simulink model "gm_HARDWARE_FRIENDLY_FSK"  (R2024a)
settings: Solver=FixedStepDiscrete  StartTime=0.0  StopTime=3.5/B  FixedStep=1/fclk  RelTol=1e-3
undefined symbols (not defined in the file or in its folder): B, DiscIntNeverNeededParam, f0, fclk
libraries: hdlsllib x3, dsphdlsigops2 x2, simulink x1
settings Model: Creator=pc  LastModifiedBy=pc
settings OptimizationCC: BlockReduction=off  ConditionallyExecuteInputs=off
settings DebuggingCC: InheritedTsInSrcMsg=none

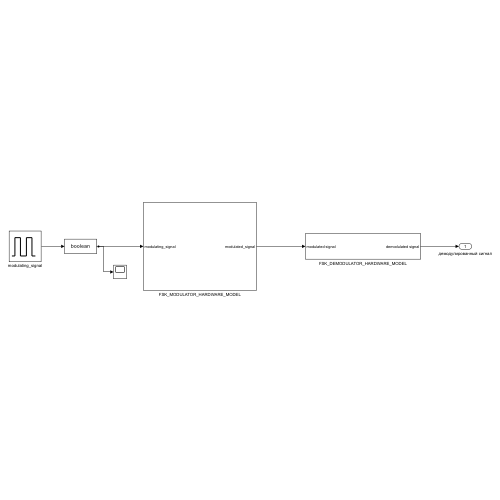
[thumbnail: Simulink's stored preview of the top-level diagram]
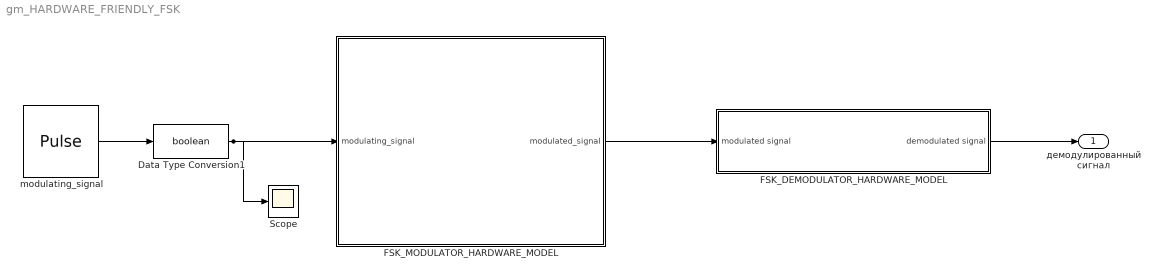
== system gm_HARDWARE_FRIENDLY_FSK ==
  Data Type Conversion1 : DataTypeConversion  OutDataTypeStr=boolean  SaturateOnIntegerOverflow=off  RndMeth=Floor
  FSK_DEMODULATOR_HARDWARE_MODEL : Subsystem
  FSK_MODULATOR_HARDWARE_MODEL : Subsystem
  Scope : Scope
  modulating_signal : DiscretePulseGenerator  PulseType=Time based  Period=2/B  PulseWidth=50
  демодулированный сигнал : Outport
  wires:
  modulating_signal/1 -> Data Type Conversion1/1
  Data Type Conversion1/1 -> FSK_MODULATOR_HARDWARE_MODEL/1(modulating_signal), Scope/1
  FSK_DEMODULATOR_HARDWARE_MODEL/1(demodulated signal) -> демодулированный сигнал/1
  FSK_MODULATOR_HARDWARE_MODEL/1(modulated_signal) -> FSK_DEMODULATOR_HARDWARE_MODEL/1(modulated signal)

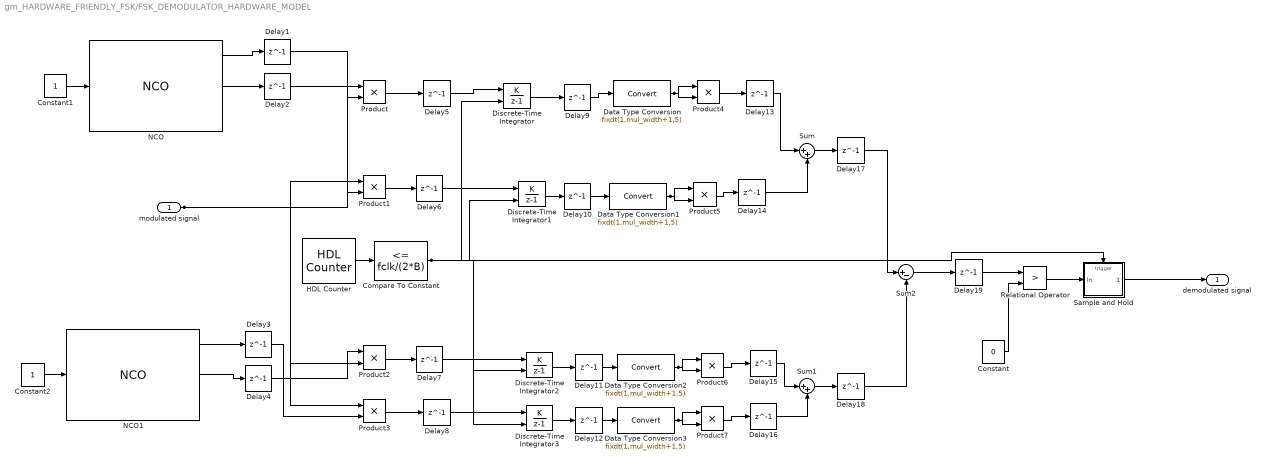
== system gm_HARDWARE_FRIENDLY_FSK/FSK_DEMODULATOR_HARDWARE_MODEL ==
  modulated signal : Inport  OutDataTypeStr=fixdt(1, 17, 15)  PortDimensions=1  SampleTime=1e-08
  Compare To Constant : simulink/Logic and Bit Operations/Compare To Constant  relop=<=  const=fclk/(2*B)  OutDataTypeStr=boolean
  Constant : Constant  Value=0  OutDataTypeStr=fixdt(1,2*mul_width+2,5)
  Constant1 : Constant  OutDataTypeStr=boolean
  Constant2 : Constant  OutDataTypeStr=boolean
  Data Type Conversion{,1..3} (4 alike) : DataTypeConversion  OutDataTypeStr=fixdt(1,mul_width+1,5)  SaturateOnIntegerOverflow=off  RndMeth=Floor
  Delay{1..19} (19 alike) : Delay  DelayLength=1  InitialCondition=0
  Discrete-Time Integrator{,1..3} (4 alike) : DiscreteIntegrator  IntegratorMethod=Accumulation: Forward Euler  ExternalReset=rising  SampleTime=-1  OutDataTypeStr=fixdt(1,sum_width,29)  ICPrevOutput=DiscIntNeverNeededParam  ICPrevScaledInput=DiscIntNeverNeededParam
  HDL Counter : hdlsllib/Sources/HDL Counter  CountType=Count limited  CountInit=0  CountStep=1  CountMax=fclk/B  CountFromType=Initial value  CountFrom=0  CountResetPort=off  CountLoadPort=off  CountEnbPort=off  CountDirPort=off  CountHitOutputPort=off  CountDataType=Unsigned  CountWordLen=30  CountFracLen=0  CountSampTime=1/fclk
  NCO : dsphdlsigops2/NCO  PhaseIncrementSource=Property  PhaseIncrement=phIncr1  PhaseOffsetSource=Property  PhaseOffset=0  DitherSource=Property  NumDitherBits=ditherBits  SamplesPerFrame=1  LUTCompress=off  ResetAction=off  Waveform=Sine and cosine  PhasePort=off  SimulateUsing=Code generation  AccumulatorWL=N  PhaseQuantization=on  NumQuantizerAccumulatorBits=Q  OutputDataType=Binary point scaling  OutputWL=16  OutputFL=15
      settings: LibrarySourceBlock=dsphdlsrcs2/NCO
  NCO1 : dsphdlsigops2/NCO  PhaseIncrementSource=Property  PhaseIncrement=phIncr2  PhaseOffsetSource=Property  PhaseOffset=0  DitherSource=Property  NumDitherBits=ditherBits  SamplesPerFrame=1  LUTCompress=off  ResetAction=off  Waveform=Sine and cosine  PhasePort=off  SimulateUsing=Code generation  AccumulatorWL=N  PhaseQuantization=on  NumQuantizerAccumulatorBits=Q  OutputDataType=Binary point scaling  OutputWL=18  OutputFL=17
      settings: LibrarySourceBlock=dsphdlsrcs2/NCO
  Product : Product  OutDataTypeStr=fixdt(1,30,29)
  Product1 : Product  OutDataTypeStr=fixdt(1,27,25)
  Product2 : Product  OutDataTypeStr=fixdt(1,27,25)
  Product3 : Product  OutDataTypeStr=fixdt(1,27,25)
  Product{4..7} (4 alike) : Product  OutDataTypeStr=fixdt(1,2*mul_width+1,5)
  Relational Operator : RelationalOperator  Operator=>  OutDataTypeStr=boolean  RndMeth=Simplest  InputSameDT=off
  Sample and Hold : Subsystem  mask(Sample and Hold){trig=Rising edge, initCond=double(0), latchinput=off}
      mask prompts: trig "dsp:DSPSignalOperationsBlockDialog:TriggerType_MP"; initCond "dsp:DSPSignalOperationsBlockDialog:InitialCondition_MP"; latchinput "dsp:DSPSignalOperationsBlockDialog:LatchInput_MP"
      mask help: dsp:DSPSignalOperationsBlockDialog:SampleAndHold_MaskDesc
      mask init:
      | initCond = double(0);
      | latchinput = double(0);
      | s = 'rising';
      | trig = double(1);
      mask Help: eval('blocksethelp');
      mask TypeOptions trig: dsp:DSPSignalOperationsBlockDialog:RisingEdge_MP | dsp:DSPSignalOperationsBlockDialog:FallingEdge_MP | dsp:DSPSignalOperationsBlockDialog:EitherEdge_MP
      mask Display: disp('S/H')
  Sum : Sum  Inputs=|++  OutDataTypeStr=fixdt(1,2*mul_width+2,5)  AccumDataTypeStr=fixdt(0,sum_width,5)
  Sum1 : Sum  Inputs=|++  OutDataTypeStr=fixdt(1,2*mul_width+2,5)  AccumDataTypeStr=fixdt(1,2*mul_width+2,5)
  Sum2 : Sum  Inputs=|+-  OutDataTypeStr=fixdt(1,2*mul_width+3,5)  AccumDataTypeStr=fixdt(1,2*mul_width+2,5)
  demodulated signal : Outport  OutDataTypeStr=boolean  SampleTime=1e-08
  wires:
  modulated signal/1 -> Product3/1, Product2/2, Product1/1, Product/2
  Compare To Constant/1 -> Sample and Hold/Trigger, Discrete-Time Integrator/2, Discrete-Time Integrator1/2, Discrete-Time Integrator2/2, Discrete-Time Integrator3/2
  Constant/1 -> Relational Operator/2
  Constant1/1 -> NCO/1
  Constant2/1 -> NCO1/1
  Data Type Conversion/1 -> Product4/2, Product4/1
  Data Type Conversion1/1 -> Product5/2, Product5/1
  Data Type Conversion2/1 -> Product6/2, Product6/1
  Data Type Conversion3/1 -> Product7/2, Product7/1
  Delay1/1 -> Product1/2
  Delay10/1 -> Data Type Conversion1/1
  Delay11/1 -> Data Type Conversion2/1
  Delay12/1 -> Data Type Conversion3/1
  Delay13/1 -> Sum/1
  Delay14/1 -> Sum/2
  Delay15/1 -> Sum1/1
  Delay16/1 -> Sum1/2
  Delay17/1 -> Sum2/1
  Delay18/1 -> Sum2/2
  Delay19/1 -> Relational Operator/1
  Delay2/1 -> Product/1
  Delay3/1 -> Product3/2
  Delay4/1 -> Product2/1
  Delay5/1 -> Discrete-Time Integrator/1
  Delay6/1 -> Discrete-Time Integrator1/1
  Delay7/1 -> Discrete-Time Integrator2/1
  Delay8/1 -> Discrete-Time Integrator3/1
  Delay9/1 -> Data Type Conversion/1
  Discrete-Time Integrator/1 -> Delay9/1
  Discrete-Time Integrator1/1 -> Delay10/1
  Discrete-Time Integrator2/1 -> Delay11/1
  Discrete-Time Integrator3/1 -> Delay12/1
  HDL Counter/1 -> Compare To Constant/1
  NCO/1 -> Delay1/1
  NCO/2 -> Delay2/1
  NCO1/1 -> Delay3/1
  NCO1/2 -> Delay4/1
  Product/1 -> Delay5/1
  Product1/1 -> Delay6/1
  Product2/1 -> Delay7/1
  Product3/1 -> Delay8/1
  Product4/1 -> Delay13/1
  Product5/1 -> Delay14/1
  Product6/1 -> Delay15/1
  Product7/1 -> Delay16/1
  Relational Operator/1 -> Sample and Hold/1(In)
  Sample and Hold/1(" ") -> demodulated signal/1
  Sum/1 -> Delay17/1
  Sum1/1 -> Delay18/1
  Sum2/1 -> Delay19/1

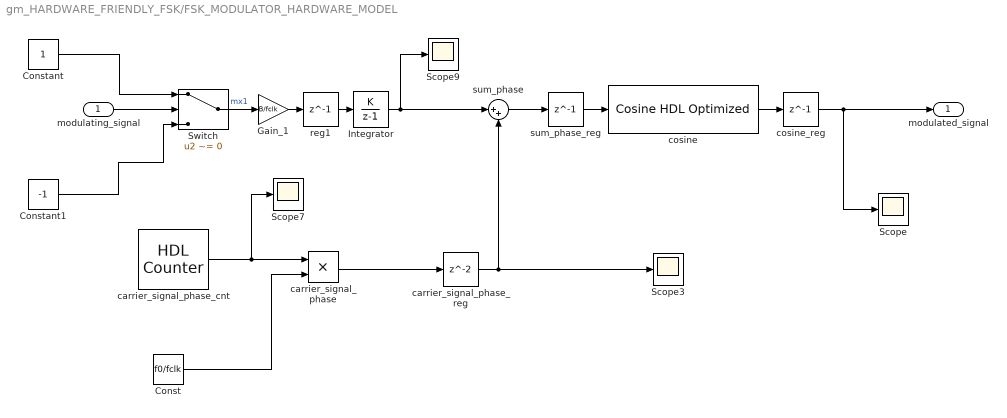
== system gm_HARDWARE_FRIENDLY_FSK/FSK_MODULATOR_HARDWARE_MODEL ==
  modulating_signal : Inport  OutDataTypeStr=boolean
  Const : Constant  Value=f0/fclk  OutDataTypeStr=fixdt(0,27,27)
  Constant : Constant  OutDataTypeStr=fixdt(1,17,15)
  Constant1 : Constant  Value=-1  OutDataTypeStr=fixdt(1,17,15)
  Gain_1 : Gain  Gain=B/fclk  ParamDataTypeStr=fixdt(0,27,27)  OutDataTypeStr=fixdt(1,28,27)  RndMeth=Round
  Integrator : DiscreteIntegrator  IntegratorMethod=Accumulation: Forward Euler  gainval=1  SampleTime=-1  OutDataTypeStr=fixdt(1,28,27)  IgnoreLimit=on  ICPrevOutput=DiscIntNeverNeededParam  ICPrevScaledInput=DiscIntNeverNeededParam
  Scope{,3,7,9} (4 alike) : Scope
  Switch : Switch  Criteria=u2 ~= 0  Threshold=0.5  OutDataTypeStr=fixdt(1,17,15)  SaturateOnIntegerOverflow=off  InputSameDT=off
  carrier_signal_phase : Product  OutDataTypeStr=fixdt(0,28,28)
  carrier_signal_phase_cnt : hdlsllib/Sources/HDL Counter  CountType=Count limited  CountInit=0  CountStep=1  CountMax=fclk/f0  CountFromType=Initial value  CountFrom=0  CountResetPort=off  CountLoadPort=off  CountEnbPort=off  CountDirPort=off  CountHitOutputPort=off  CountDataType=Unsigned  CountWordLen=16  CountFracLen=0  CountSampTime=1/fclk
  carrier_signal_phase_reg : Delay  InitialCondition=0
  cosine : hdlsllib/Lookup Tables/Cosine HDL Optimized  OutputFormula=cos(2*pi*u)  NumDataPoints=2048  TableDataTypeStr=fixdt(1,16,15)  SimulateLUTROMDelay=on
  cosine_reg : Delay  DelayLength=1  InitialCondition=0
  reg1 : Delay  DelayLength=1  InitialCondition=0
  sum_phase : Sum  Inputs=|++  AccumDataTypeStr=fixdt(1,29,28)
  sum_phase_reg : Delay  DelayLength=1  InitialCondition=0
  modulated_signal : Outport
  wires:
  cosine_reg/1 -> modulated_signal/1, Scope/1
  cosine/1 -> cosine_reg/1
  carrier_signal_phase_reg/1 -> sum_phase/2, Scope3/1
  carrier_signal_phase/1 -> carrier_signal_phase_reg/1
  sum_phase/1 -> sum_phase_reg/1
  sum_phase_reg/1 -> cosine/1
  reg1/1 -> Integrator/1
  Gain_1/1 -> reg1/1
  Integrator/1 -> sum_phase/1, Scope9/1
  Switch/1 -> Gain_1/1  "mx1"
  carrier_signal_phase_cnt/1 -> carrier_signal_phase/1, Scope7/1
  Const/1 -> carrier_signal_phase/2
  Constant1/1 -> Switch/3
  Constant/1 -> Switch/1
  modulating_signal/1 -> Switch/2

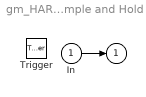
== system gm_HARDWARE_FRIENDLY_FSK/FSK_DEMODULATOR_HARDWARE_MODEL/Sample and Hold ==
  In : Inport  OutDataTypeStr=boolean
  Trigger : TriggerPort  VariantControl=(inherit)  OutDataTypeStr=boolean
  " " : Outport  InitialOutput=0
  wires:
  In/1 -> " "/1
